simulink model "Tanks_Template"  (R2021b)
settings: Solver=ode4  StartTime=0.0  StopTime=inf  FixedStep=0.001  RelTol=1e-3
PostLoadFcn:
  | qc_set_target_type(getConfigSet(bdroot, 'QUARC Default Target Configuration'));
values from neighbouring files (symbols this model uses):
  A_sys = [-k1,  0 ... (first row only)    [test1.m]
  B_sys = gain_pump * [(gamma_1) / S ... (first row only)    [test1.m]
  C_sys = eye(2,2)    [test1.m]
  D_sys = [0 ... (first row only)    [test1.m]
  gain_1 = theta_LLS_1(1)    [test1.m]
  gain_2 = theta_LLS_2(1)    [test1.m]
  h1_eq = q^2 * gamma_1^2 / (2*g*A_D1^2)    (= 13.8803423879)    [test1.m]
  h2_eq = q^2 / (2*g*A_D2^2)    (= 13.6625202321)    [test1.m]
  Ka = place(A_sys, B_sys, wanted_poles)    [test1.m]
  Kff = -inv([0 1]*inv(A_sys - B_sys*Ka)*B_sys)    [test1.m]
  offset_1 = offset_1+mean(final_offset.data(3, 45e2:50e2))    [test1.m]
  offset_2 = offset_2+mean(final_offset.data(2, 45e2:50e2))    [test1.m]
undefined symbols (not defined in the file or in its folder): HIL
libraries: quarc_library x4
settings Model: SimulationMode=external  ExtModeTrigDuration=30000  Creator=MLevis  LastModifiedBy=user
settings SolverCC: AlgebraicLoopSolver=TrustRegion  PositivePriorityOrder=on
settings DataIOCC: LimitDataPoints=on  SaveFormat=Array  SignalLoggingSaveFormat=ModelDataLogs  ReturnWorkspaceOutputs=off
settings OptimizationCC: ExpressionDepthLimit=2147483647  InitFltsAndDblsToZero=on
settings DebuggingCC: SaveWithParameterizedLinksMsg=none  MergeDetectMultiDrivingBlocksExec=none  SolverPrmCheckMsg=warning  MultiTaskDSMMsg=warning  MultiTaskCondExecSysMsg=none  MultiTaskRateTransMsg=warning  FcnCallInpInsideContextMsg=warning  StateNameClashWarn=warning  SFUnexpectedBacktrackingDiag=warning  SFNoUnconditionalDefaultTransitionDiag=warning  SFExecutionAtInitializationDiag=none  ArithmeticOperatorsInVariantConditions=warning
settings ModelReferenceCC: PropagateSignalLabelsOutOfModel=off
settings SFSimCC: SimUseLocalCustomCode=off  CustomCodeUndefinedFunction=UseInterfaceOnly
settings RTWCC: Description=QUARC Win64 Target Using Toolchain  SystemTargetFile=quarc_win64.tlc  TemplateMakefile=quarc_default_tmf  RTWUseLocalCustomCode=off  Toolchain=QUARC win64 | nmake (64-bit Windows)  BuildConfiguration=Faster Runs
settings CodeAppCC: StateflowObjectComments=on
settings STFCustomTargetCC: ConcurrentExecutionCompliant=on  UseToolchainInfoCompliant=on  SystemTargetFile=quarc_win64.tlc
settings GRTTargetCC: TargetLangStandard=C89/C90 (ANSI)  ParMdlRefBuildCompliant=off  CompOptLevelCompliant=off  CombineOutputUpdateFcns=off  MatFileLogging=off  CPPClassGenCompliant=off  GRTInterface=on  ExtMode=on  ExtModeMexFile=quarc_comm
settings ConfigComp: CovMetricSettings=dw  CovSaveCumulativeToWorkspaceVar=on  CovSaveSingleToWorkspaceVar=on  CovExternalEMLEnable=off

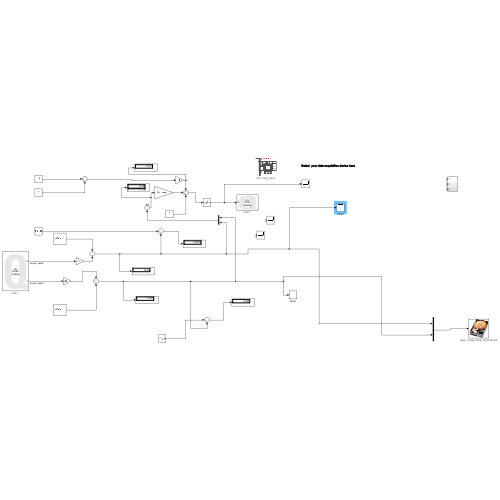
[thumbnail: Simulink's stored preview of the top-level diagram]
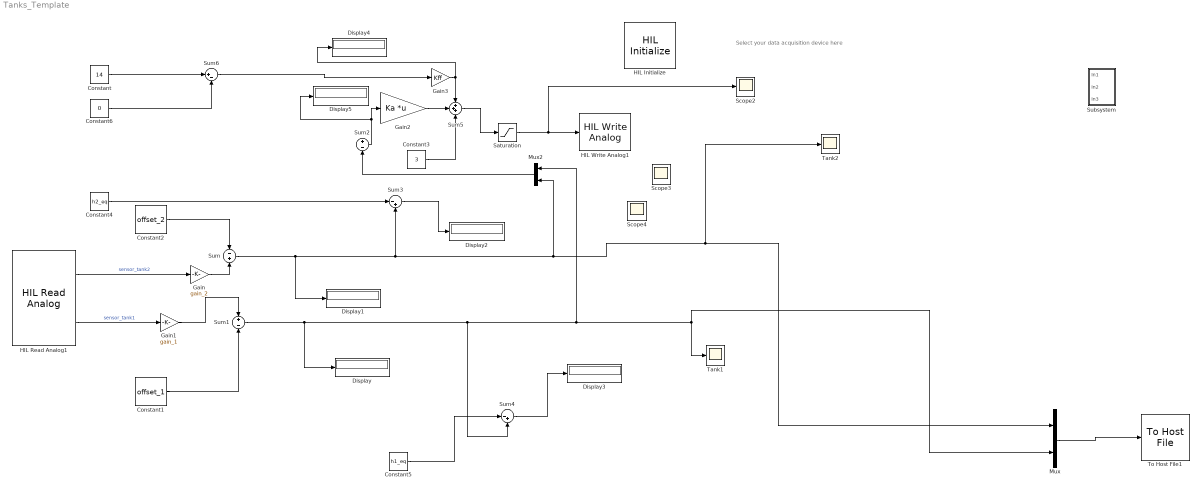
== system Tanks_Template ==
  note: Select your data acquisition device here
  Constant : Constant  Value=14
  Constant1 : Constant  Value=offset_1
  Constant2 : Constant  Value=offset_2
  Constant3 : Constant  Value=3
  Constant4 : Constant  Value=h2_eq
  Constant5 : Constant  Value=h1_eq
  Constant6 : Constant  Value=0
  Display{,1..5} (6 alike) : Display
  Gain : Gain  Gain=gain_2
  Gain1 : Gain  Gain=gain_1
  Gain2 : Gain  Gain=Ka  Multiplication=Matrix(K*u) (u vector)
  Gain3 : Gain  Gain=Kff
  HIL Initialize : quarc_library/Data Acquisition/Generic/Configuration/HIL Initialize  object_name=HIL-1  board_type=q8_usb  board_number=0  board_options=update_rate=normal;decimation=1  exclusive=off  active=off  hardware_clocks=[0:2]  clock_modes=[]  initial_clock_frequencies=[]  set_clock_params_at_start=off  set_clock_params_at_switch_in=off  set_clock_frequencies_at_start=off  set_clock_frequencies_at_switch_in=off  analog_input_channels=[0:7]  analog_input_configurations=[]  analog_input_maximums=10  analog_input_minimums=-10  set_analog_input_params_at_start=on  set_analog_input_params_at_switch_in=off  analog_output_channels=[0:7]  analog_output_maximums=10  analog_output_minimums=-10  initial_analog_outputs=[0]  final_analog_outputs=[0]  watchdog_analog_outputs=0  set_analog_output_params_at_start=on  set_analog_output_params_at_switch_in=off  set_analog_outputs_at_start=on  set_analog_outputs_at_switch_in=off  set_analog_outputs_at_terminate=on  set_analog_outputs_at_switch_out=off  set_analog_outputs_on_watchdog=off  digital_input_channels=[]  digital_output_channels=[]  digital_output_configuration=[]  initial_digital_outputs=[1]  final_digital_outputs=[1]  watchdog_digital_outputs=[1]  set_digital_output_params_at_start=off  set_digital_output_params_at_switch_in=off  set_digital_outputs_at_start=on  set_digital_outputs_at_switch_in=off  set_digital_outputs_at_terminate=on  set_digital_outputs_at_switch_out=off  set_digital_outputs_on_watchdog=off  encoder_channels=[0:7]  quadrature=[4]  encoder_filter_frequency=[]  initial_encoder_counts=[0]  set_encoder_params_at_start=on  set_encoder_params_at_switch_in=off  set_encoder_counts_at_start=on  set_encoder_counts_at_switch_in=off  pwm_channels=[0:7]  pwm_modes=0  pwm_frequency=99.532799999999995e6/4095  pwm_configuration=[0]  pwm_alignment=[0]  pwm_polarity=[1]  pwm_leading_deadband=[0]  pwm_trailing_deadband=[0]  initial_pwm_outputs=[0]  final_pwm_outputs=[0]  watchdog_pwm_outputs=[0]  set_pwm_params_at_start=on  set_pwm_params_at_switch_in=off  set_pwm_outputs_at_start=on  set_pwm_outputs_at_switch_in=off  set_pwm_outputs_at_terminate=on  set_pwm_outputs_at_switch_out=off  set_pwm_outputs_on_watchdog=off  other_output_channels=[]  initial_other_outputs=[]  final_other_outputs=[]  watchdog_other_outputs=[]  set_other_outputs_at_start=off  set_other_outputs_at_switch_in=off  set_other_outputs_at_terminate=off  set_other_outputs_at_switch_out=off  set_other_outputs_on_watchdog=off
  HIL Read Analog1 : quarc_library/Data Acquisition/Generic/Immediate I//O/HIL Read Analog  object_name=HIL-1  channels=[0:1]  sample_time=0.01  active=on  vector_output=off
  HIL Write Analog1 : quarc_library/Data Acquisition/Generic/Immediate I//O/HIL Write Analog  object_name=HIL-1  channels=[0]  sample_time=-1  active=off  vector_input=off
  Mux : Mux  Inputs=2
  Mux2 : Mux  Inputs=2
  Saturation : Saturate  UpperLimit=12  LowerLimit=0
  Scope2 : Scope
  Scope3 : Scope
  Scope4 : Scope
  Subsystem : Subsystem
  Sum : Sum  Inputs=-+
  Sum1 : Sum  Inputs=+-
  Sum2 : Sum  Inputs=+-
  Sum3 : Sum  Inputs=|-+
  Sum4 : Sum  Inputs=|-+
  Sum5 : Sum  Inputs=+++
  Sum6 : Sum  Inputs=|+-
  Tank1 : Scope
  Tank2 : Scope
  To Host File1 : quarc_library/Sinks/To Host/To Host File  file_name=Data_%{date}_%{time}.mat  variable_name=data  decimation=1  sample_time=0.01  file_format=MAT-file v.4  options=No header or footer  append=off  final_file_name=Data_19-Mar-2026_18-45-38.mat  bitrate=2000000
  wires:
  Mux/1 -> To Host File1/1
  HIL Read Analog1/1 -> Gain/1  "sensor_tank2"
  Gain/1 -> Sum/2
  HIL Read Analog1/2 -> Gain1/1  "sensor_tank1"
  Gain1/1 -> Sum1/1
  Constant1/1 -> Sum1/2
  Constant2/1 -> Sum/1
  Gain2/1 -> Sum5/2
  Sum1/1 -> Display/1, Mux2/1, Mux/2, Tank1/1, Sum4/2
  Saturation/1 -> Scope2/1, HIL Write Analog1/1
  Constant4/1 -> Sum3/1
  Constant5/1 -> Sum4/1
  Sum3/1 -> Display2/1
  Sum4/1 -> Display3/1
  Mux2/1 -> Sum2/2
  Sum/1 -> Display1/1, Sum3/2, Mux2/2, Tank2/1, Mux/1
  Constant/1 -> Sum6/1
  Sum5/1 -> Saturation/1
  Constant3/1 -> Sum5/3
  Constant6/1 -> Sum6/2
  Sum6/1 -> Gain3/1
  Sum2/1 -> Display5/1, Gain2/1
  Gain3/1 -> Sum5/1, Display4/1

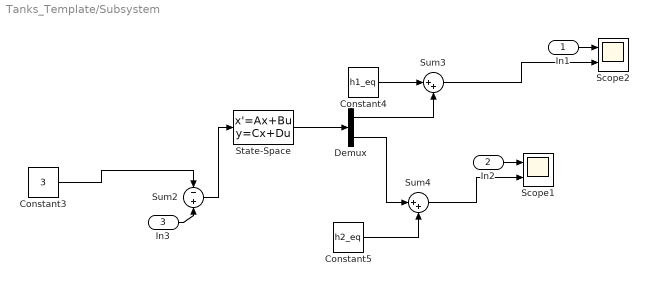
== system Tanks_Template/Subsystem ==
  In1 : Inport
  In2 : Inport  Port=2
  In3 : Inport  Port=3
  Constant3 : Constant  Value=3
  Constant4 : Constant  Value=h1_eq
  Constant5 : Constant  Value=h2_eq
  Demux : Demux  Outputs=2
  Scope1 : Scope  NumInputPorts=2
  Scope2 : Scope  NumInputPorts=2
  State-Space : StateSpace  A=A_sys  B=B_sys  C=C_sys  D=D_sys  InitialCondition=0
  Sum2 : Sum  Inputs=-+
  Sum3 : Sum  Inputs=|++
  Sum4 : Sum  Inputs=|++
  wires:
  Sum2/1 -> State-Space/1
  Sum4/1 -> Scope1/2
  Demux/1 -> Sum3/2
  Constant5/1 -> Sum4/2
  Sum3/1 -> Scope2/2
  In1/1 -> Scope2/1
  In3/1 -> Sum2/2
  Demux/2 -> Sum4/1
  State-Space/1 -> Demux/1
  Constant3/1 -> Sum2/1
  Constant4/1 -> Sum3/1
  In2/1 -> Scope1/1
